simulink model "test_mambo_open_loop"  (R2022b)
settings: Solver=VariableStepAuto  StartTime=0.0  StopTime=10.0  RelTol=1e-3
values from neighbouring files (symbols this model uses):
  Ad = MLD.A    [parrot_mambo_main.m]
  Bd = MLD.B    [parrot_mambo_main.m]
  Cd = MLD.C    [parrot_mambo_main.m]
  Dd = MLD.D    [parrot_mambo_main.m]
  Ts = 0.01    [parrot_mambo_main.m]
settings Model: Creator=phatdo  LastModifiedBy=phatdo
settings DataIOCC: ReturnWorkspaceOutputs=off

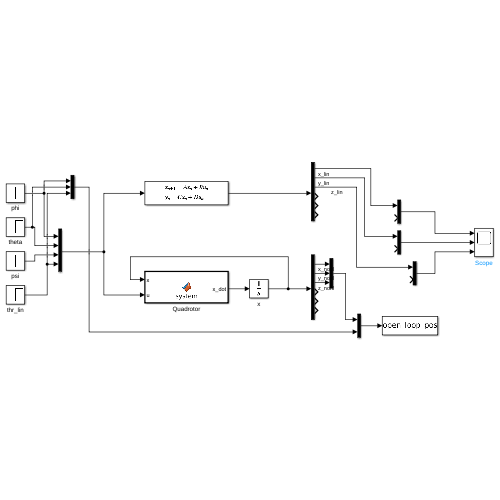
[thumbnail: Simulink's stored preview of the top-level diagram]
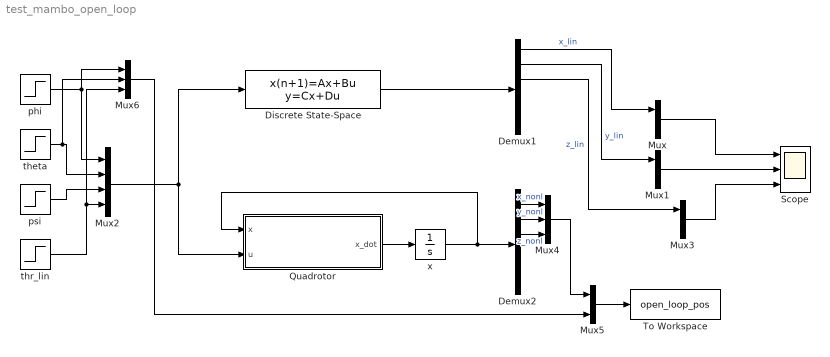
== system test_mambo_open_loop ==
  Demux1 : Demux  Outputs=6
  Demux2 : Demux  Outputs=6
  Discrete State-Space : DiscreteStateSpace  A=Ad  B=Bd  C=Cd  D=Dd  SampleTime=Ts
  Mux{,1,3,5} (4 alike) : Mux  Inputs=2
  Mux2 : Mux
  Mux4 : Mux  Inputs=3
  Mux6 : Mux  Inputs=3
  Quadrotor : MATLAB Function  TreatAsAtomicUnit=on
  Scope : Scope  NumInputPorts=3
  To Workspace : ToWorkspace  VariableName=open_loop_pos  SaveFormat=Timeseries  SampleTime=-1
  phi : Step  Time=0  After=0.05  SampleTime=Ts
  psi : Step  Time=0  After=0  SampleTime=Ts
  theta : Step  Time=0  After=0.05  SampleTime=Ts
  thr_lin : Step  Time=0  After=0.5  SampleTime=Ts
  x : Integrator
  wires:
  phi/1 -> Mux2/1, Mux6/1
  theta/1 -> Mux6/2, Mux2/2
  psi/1 -> Mux2/3
  Quadrotor/1(x_dot) -> x/1
  x/1 -> Quadrotor/1(x), Demux2/1
  Discrete State-Space/1 -> Demux1/1
  Demux1/1 -> Mux/1  "x_lin"
  Demux1/2 -> Mux1/1  "y_lin"
  Demux1/3 -> Mux3/1  "z_lin"
  Mux/1 -> Scope/1
  Mux1/1 -> Scope/2
  Mux3/1 -> Scope/3
  thr_lin/1 -> Mux6/3, Mux2/4
  Mux2/1 -> Discrete State-Space/1, Quadrotor/2(u)
  Demux2/1 -> Mux4/1  "x_nonl"
  Demux2/2 -> Mux4/2  "y_nonl"
  Demux2/3 -> Mux4/3  "z_nonl"
  Mux4/1 -> Mux5/1
  Mux6/1 -> Mux5/2
  Mux5/1 -> To Workspace/1

== matlab function test_mambo_open_loop/Quadrotor ==
  data: x input; u input; x_dot output
function x_dot = system(x,u)
%% Init
% x = [x y z x_dot y_dot z_dot]
% u = [phi theta psi delta_T]
x_dot = zeros(6,1);
m = 1.0;
g = 9.81;

%% Output
c_phi   = cos(u(1));
c_theta = cos(u(2));
c_psi   = cos(u(3));
s_phi   = sin(u(1));
s_theta = sin(u(2));
s_psi   = sin(u(3));
deltaT = u(4);

T = deltaT + m*g;

x_dot(1) = x(4);
x_dot(2) = x(5);
x_dot(3) = x(6);
x_dot(4) = (c_phi*s_theta*c_psi + s_phi*s_psi)*T/m;
x_dot(5) = (c_phi*s_theta*s_psi - s_phi*c_psi)*T/m;
x_dot(6) = -g + c_phi*c_theta*T/m;

end
